simulink model "UKF_XY"  (R2020b)
settings: Solver=ode45  StartTime=0.0  StopTime=180  FixedStep=1e-7  RelTol=1e-4  AbsTol=1e-4  EnableMultiTasking=on
libraries: simulink x2
settings Model: Creator=André  LastModifiedBy=Andre
settings SolverCC: AutoScaleAbsTol=off  ConsecutiveZCsStepRelTol=100*128*eps  ShapePreserveControl=EnableAll  ZeroCrossControl=EnableAll  AutoInsertRateTranBlk=on
settings DataIOCC: LimitDataPoints=on  SaveFormat=Array  SignalLoggingSaveFormat=ModelDataLogs  ReturnWorkspaceOutputs=off
settings OptimizationCC: ExpressionDepthLimit=2147483647  LifeSpan=inf
settings DebuggingCC: UnderspecifiedInitializationDetection=Classic  MergeDetectMultiDrivingBlocksExec=none  SolverPrmCheckMsg=warning  FcnCallInpInsideContextMsg=warning  StateNameClashWarn=warning  SFUnexpectedBacktrackingDiag=warning  SFNoUnconditionalDefaultTransitionDiag=warning  SFExecutionAtInitializationDiag=none  ArithmeticOperatorsInVariantConditions=warning
settings HardwareCC: ProdBitPerPointer=32  ProdBitPerSizeT=32  ProdBitPerPtrDiffT=32  ProdLargestAtomicFloat=None  ProdIntDivRoundTo=Undefined  ProdEndianess=Unspecified  ProdWordSize=32  ProdHWDeviceType=32-bit Generic
settings ModelReferenceCC: PropagateSignalLabelsOutOfModel=off
settings SFSimCC: SimUseLocalCustomCode=off  SimParseCustomCode=off  CustomCodeUndefinedFunction=UseInterfaceOnly
settings RTWCC: RTWUseLocalCustomCode=off
settings CodeAppCC: StateflowObjectComments=on
settings GRTTargetCC: TargetLangStandard=C89/C90 (ANSI)  CombineOutputUpdateFcns=off  GRTInterface=on
settings ConfigComp: CovMetricSettings=dw  CovSaveCumulativeToWorkspaceVar=on  CovSaveSingleToWorkspaceVar=on  CovExternalEMLEnable=off

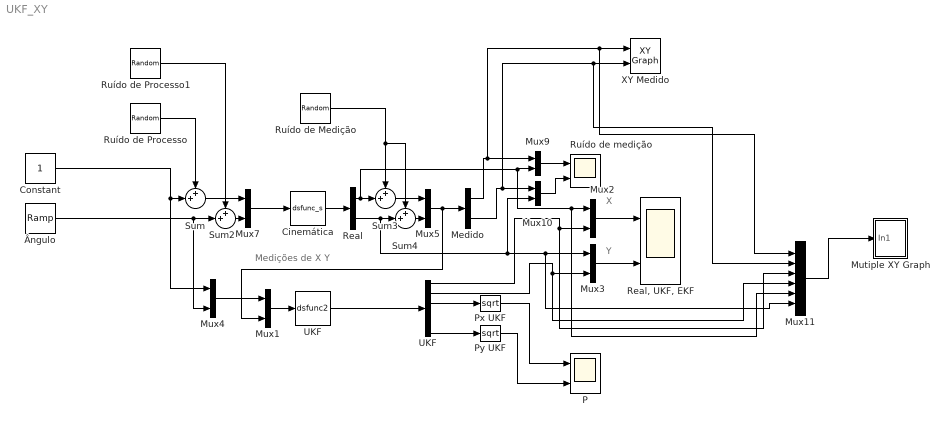
== system UKF_XY ==
  note: Y
  note: X
  note: Medições de X Y
  Cinemática : S-Function  FunctionName=dsfunc_s  Parameters=[0 0]  SFunctionDeploymentMode=off  EnableBusSupport=off
  Constant : Constant
  Medido : Demux  Outputs=2
  Mutiple XY Graph : Subsystem  mask(Mutiple XY Graph){number_of_trajectories=3, axis_limits=[-200 200 -200 200], sample_time=0.1}
      mask prompts: number_of_trajectories "Number of Trajectories"; axis_limits "Axis Limits"; sample_time "Sample Time"
      mask Display: plot([.05 .95 .95 .05 .05],[.45 .45 .95 .95 .45], 0.5+cos(0:0.1:2*pi)*0.3,0.7+sin(0:0.1:2*pi)*0.2)
  Mux{1..5,7,9..10} (8 alike) : Mux  Inputs=2
  Mux11 : Mux  Inputs=6
  P : Scope  NumInputPorts=2
  Px UKF : Sqrt  SaturateOnIntegerOverflow=on
  Py UKF : Sqrt  SaturateOnIntegerOverflow=on
  Real : Demux  Outputs=2
  "Real, UKF, EKF" : Scope  NumInputPorts=2
  Ruído de Medição : RandomNumber  SampleTime=0.01
  Ruído de Processo : RandomNumber  SampleTime=0.01
  Ruído de Processo1 : RandomNumber  Variance=0.1  SampleTime=1
  Ruído de medição : Scope  NumInputPorts=2
  Sum{,2..4} (4 alike) : Sum  Inputs=++|
  UKF : S-Function  FunctionName=dsfunc2  Parameters=[-20 -20 100 0 0 100]  SFunctionDeploymentMode=off  EnableBusSupport=off
  "UKF  " : Demux  Outputs=6
  XY Medido : simulink/Sinks/XY Graph  xmin=-200  xmax=200  ymin=-200  ymax=200  st=-1
  Ângulo : simulink/Sources/Ramp  slope=0.1/pi  start=0  InitialOutput=0
  wires:
  Medido/1 -> Mux11/1, XY Medido/1, Mux9/1
  Medido/2 -> Mux11/2, XY Medido/2, Mux10/1
  Mux1/1 -> UKF/1
  UKF/1 -> "UKF  "/1
  "UKF  "/2 -> Mux11/4, Mux3/2
  Ruído de Processo/1 -> Sum/1
  Mux7/1 -> Cinemática/1
  Mux5/1 -> Mux1/2, Medido/1
  "UKF  "/1 -> Mux11/3, Mux2/2
  Mux2/1 -> "Real, UKF, EKF"/1
  Mux3/1 -> "Real, UKF, EKF"/2
  "UKF  "/3 -> Px UKF/1
  "UKF  "/6 -> Py UKF/1
  Sum2/1 -> Mux7/2
  Constant/1 -> Mux4/1, Sum/2
  Sum/1 -> Mux7/1
  Mux4/1 -> Mux1/1
  Cinemática/1 -> Real/1
  Sum3/1 -> Mux5/1
  Ruído de Medição/1 -> Sum3/1, Sum4/1
  Real/2 -> Mux11/6, Mux3/1, Mux10/2, Sum4/2
  Sum4/1 -> Mux5/2
  Real/1 -> Mux11/5, Mux2/1, Mux9/2, Sum3/2
  Px UKF/1 -> P/1
  Mux10/1 -> Ruído de medição/2
  Mux9/1 -> Ruído de medição/1
  Mux11/1 -> Mutiple XY Graph/1(In1)
  Ângulo/1 -> Mux4/2, Sum2/2
  Ruído de Processo1/1 -> Sum2/1
  Py UKF/1 -> P/2

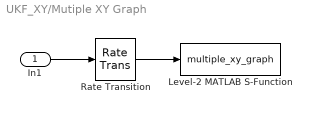
== system UKF_XY/Mutiple XY Graph ==
  In1 : Inport
  Level-2 MATLAB S-Function : M-S-Function  FunctionName=multiple_xy_graph  Parameters=number_of_trajectories,axis_limits
  Rate Transition : RateTransition  OutPortSampleTime=sample_time
  wires:
  In1/1 -> Rate Transition/1
  Rate Transition/1 -> Level-2 MATLAB S-Function/1
